simulink model "sim3"  (R2024a)
settings: Solver=FixedStepAuto  StartTime=0.0  StopTime=10.0  FixedStep=1  RelTol=1e-3
settings Model: Creator=alexe  LastModifiedBy=alexe

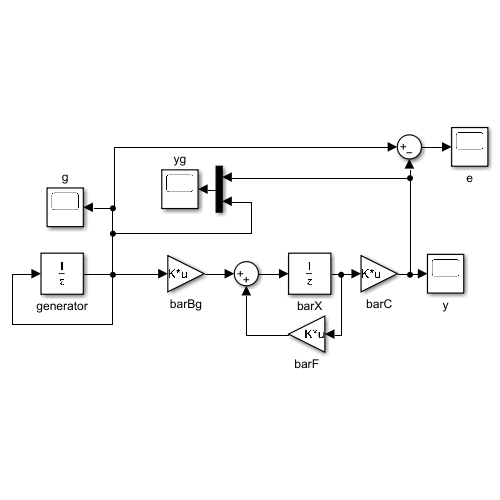
[thumbnail: Simulink's stored preview of the top-level diagram]
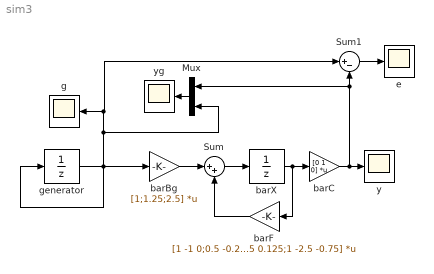
== system sim3 ==
  Mux : Mux  Inputs=2
  Sum : Sum  Inputs=|++
  Sum1 : Sum  Inputs=|+-
  barBg : Gain  Gain=[1;1.25;2.5]  Multiplication=Matrix(K*u)
  barC : Gain  Gain=[0 1 0]  Multiplication=Matrix(K*u)
  barF : Gain  Gain=[1 -1 0;0.5 -0.25 0.125;1 -2.5 -0.75]  Multiplication=Matrix(K*u)
  barX : UnitDelay  InitialCondition=[0;1;0]  SampleTime=-1  HasFrameUpgradeWarning=on
  e : Scope
  g : Scope
  generator : UnitDelay  InitialCondition=2.12  SampleTime=-1  HasFrameUpgradeWarning=on
  y : Scope
  yg : Scope
  wires:
  generator/1 -> barBg/1, Mux/2, Sum1/1, g/1, generator/1
  barBg/1 -> Sum/1
  Sum/1 -> barX/1
  barF/1 -> Sum/2
  barX/1 -> barF/1, barC/1
  barC/1 -> Mux/1, Sum1/2, y/1
  Sum1/1 -> e/1
  Mux/1 -> yg/1
